simulink model "sinepwm"  (R2018a)
settings: Solver=VariableStepAuto  StartTime=0.0  StopTime=10  RelTol=1e-3
libraries: powerlib x21, simulink x7, powerlib_meascontrol x1
settings Model: Creator=Emre Deniz  LastModifiedBy=Emre Deniz
settings SolverCC: ZeroCrossAlgorithm=Adaptive
settings DebuggingCC: MaxConsecutiveZCsMsg=none

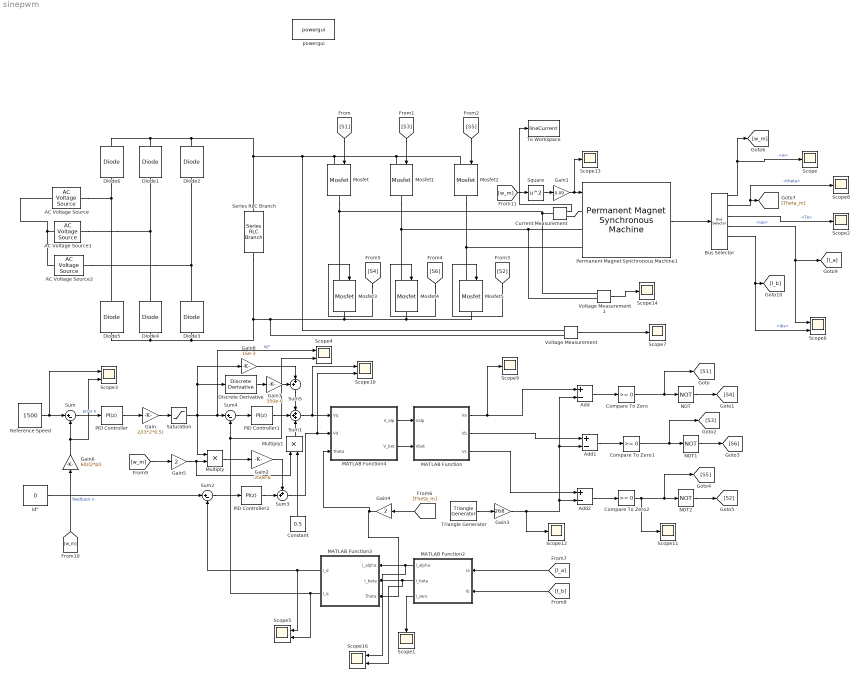
== system sinepwm ==
  AC Voltage Source : powerlib/Electrical Sources/AC Voltage Source  Amplitude=230*sqrt(2)  Phase=0  Frequency=50  SampleTime=0  Measurements=None  BusType=swing  Pref=10e3  Qref=0  Qmin=-inf  Qmax=+inf
  AC Voltage Source1 : powerlib/Electrical Sources/AC Voltage Source  Amplitude=230*sqrt(2)  Phase=-120  Frequency=50  SampleTime=0  Measurements=None  BusType=swing  Pref=10e3  Qref=0  Qmin=-inf  Qmax=+inf
  AC Voltage Source2 : powerlib/Electrical Sources/AC Voltage Source  Amplitude=230*sqrt(2)  Phase=+120  Frequency=50  SampleTime=0  Measurements=None  BusType=swing  Pref=10e3  Qref=0  Qmin=-inf  Qmax=+inf
  Add : Sum  Inputs=+-
  Add1 : Sum  Inputs=+-
  Add2 : Sum  Inputs=+-
  Bus Selector : BusSelector  OutputSignals=w,theta,Te,ias,ibs,ics
  Compare To Zero : simulink/Logic and Bit Operations/Compare To Zero  relop=>=  OutDataTypeStr=boolean
  Compare To Zero1 : simulink/Logic and Bit Operations/Compare To Zero  relop=>=  OutDataTypeStr=boolean
  Compare To Zero2 : simulink/Logic and Bit Operations/Compare To Zero  relop=>=  OutDataTypeStr=boolean
  Constant : Constant  Value=0.5
  Current Measurement : powerlib/Measurements/Current Measurement  PhasorSimulation=off  OutputType=Complex  PSBequivalent=0
  Diode{1..6} (6 alike) : powerlib/Power Electronics/Diode  Ron=0.001  Lon=0  Vf=0.8  IC=0  UseSnubber=0  Rs=500  Cs=250e-9  Measurements=off
  Discrete Derivative : simulink/Quick Insert/Discrete/Discrete Derivative  gainval=1.0  ICPrevScaledInput=0.0  OutMin=[]  OutMax=[]  OutDataType=fixdt(1, 16)  OutScaling=2^-10  DoSatur=off
      settings: SourceProductName=Simulink  SourceProductBaseCode=SL
  Gain : Gain  Gain=2/(3*2*0.5)
  Gain1 : Gain  Gain=0.09
  Gain2 : Gain  Gain=-350e-6
  Gain3 : Gain  Gain=268
  Gain4 : Gain  Gain=2
  Gain5 : Gain  Gain=2
  Gain6 : Gain  Gain=60/(2*pi)
  Gain7 : Gain  Gain=350e-6
  Gain8 : Gain  Gain=16e-3
  "Id\" " : Constant  Value=0
  MATLAB Function : MATLAB Function  TreatAsAtomicUnit=on
  MATLAB Function2 : MATLAB Function  TreatAsAtomicUnit=on
  MATLAB Function3 : MATLAB Function  TreatAsAtomicUnit=on
  MATLAB Function4 : MATLAB Function  TreatAsAtomicUnit=on
  Mosfet{,1..5} (6 alike) : powerlib/Power Electronics/Mosfet  Ron=0  Lon=0  Rd=0  Vfd=0  IC=0  Rs=1e9  Cs=inf  Measurements=off
  Multiply : Product
  Multiply1 : Product
  NOT : Logic  Operator=NOT  IconShape=distinctive  AllPortsSameDT=off  OutDataTypeStr=boolean
  NOT1 : Logic  Operator=NOT  IconShape=distinctive  AllPortsSameDT=off  OutDataTypeStr=boolean
  NOT2 : Logic  Operator=NOT  IconShape=distinctive  AllPortsSameDT=off  OutDataTypeStr=boolean
  PID Controller : simulink/Continuous/PID Controller  Controller=PI  TimeDomain=Discrete-time  SampleTime=-1  IntegratorMethod=Forward Euler  FilterMethod=Forward Euler  Form=Parallel  UseFilter=on  ControllerParametersSource=internal  P=200  I=1  D=0  N=100  InitialConditionSource=internal  InitialConditionForIntegrator=0  InitialConditionForFilter=0  ExternalReset=none  LimitOutput=off  UpperSaturationLimit=inf  LowerSaturationLimit=-inf  LinearizeAsGain=on  AntiWindupMode=none  Kb=1  TrackingMode=off  Kt=1  PParamMin=[]  PParamMax=[]  IParamMin=[]  IParamMax=[]  DParamMin=[]  DParamMax=[]  NParamMin=[]  NParamMax=[]  KbParamMin=[]  KbParamMax=[]  KtParamMin=[]  KtParamMax=[]  POutMin=[]  POutMax=[]  IOutMin=[]  IOutMax=[]  DOutMin=[]  DOutMax=[]  NOutMin=[]  NOutMax=[]  KbOutMin=[]  KbOutMax=[]  KtOutMin=[]  KtOutMax=[]  IntegratorOutMin=[]  IntegratorOutMax=[]  FilterOutMin=[]  FilterOutMax=[]  SumOutMin=[]  SumOutMax=[]  SumI1OutMin=[]  SumI1OutMax=[]  SumI2OutMin=[]  SumI2OutMax=[]  SumI3OutMin=[]  SumI3OutMax=[]  SumDOutMin=[]  SumDOutMax=[]  SaturationOutMin=[]  SaturationOutMax=[]  IntegratorContinuousStateAttributes=''  IntegratorStateMustResolveToSignalObject=off  IntegratorRTWStateStorageClass=Auto  FilterContinuousStateAttributes=''  FilterStateMustResolveToSignalObject=off  FilterRTWStateStorageClass=Auto  DifferentiatorICPrevScaledInput=0  DifferentiatorOutMin=[]  DifferentiatorOutMax=[]  FilterDiffOutCoefMin=[]  FilterDiffOutCoefMax=[]  SumDenOutMin=[]  SumDenOutMax=[]  SumNumOutMin=[]  SumNumOutMax=[]  ReciprocalOutMin=[]  ReciprocalOutMax=[]  DivideOutMin=[]  DivideOutMax=[]  TunerSelectOption=Transfer Function Based (PID Tuner App)
  PID Controller1 : simulink/Continuous/PID Controller  Controller=PI  TimeDomain=Discrete-time  SampleTime=-1  IntegratorMethod=Forward Euler  FilterMethod=Forward Euler  Form=Parallel  UseFilter=on  ControllerParametersSource=internal  P=0.01  I=50  D=0  N=100  InitialConditionSource=internal  InitialConditionForIntegrator=0  InitialConditionForFilter=0  ExternalReset=none  LimitOutput=off  UpperSaturationLimit=inf  LowerSaturationLimit=-inf  LinearizeAsGain=on  AntiWindupMode=none  Kb=1  TrackingMode=off  Kt=1  PParamMin=[]  PParamMax=[]  IParamMin=[]  IParamMax=[]  DParamMin=[]  DParamMax=[]  NParamMin=[]  NParamMax=[]  KbParamMin=[]  KbParamMax=[]  KtParamMin=[]  KtParamMax=[]  POutMin=[]  POutMax=[]  IOutMin=[]  IOutMax=[]  DOutMin=[]  DOutMax=[]  NOutMin=[]  NOutMax=[]  KbOutMin=[]  KbOutMax=[]  KtOutMin=[]  KtOutMax=[]  IntegratorOutMin=[]  IntegratorOutMax=[]  FilterOutMin=[]  FilterOutMax=[]  SumOutMin=[]  SumOutMax=[]  SumI1OutMin=[]  SumI1OutMax=[]  SumI2OutMin=[]  SumI2OutMax=[]  SumI3OutMin=[]  SumI3OutMax=[]  SumDOutMin=[]  SumDOutMax=[]  SaturationOutMin=[]  SaturationOutMax=[]  IntegratorContinuousStateAttributes=''  IntegratorStateMustResolveToSignalObject=off  IntegratorRTWStateStorageClass=Auto  FilterContinuousStateAttributes=''  FilterStateMustResolveToSignalObject=off  FilterRTWStateStorageClass=Auto  DifferentiatorICPrevScaledInput=0  DifferentiatorOutMin=[]  DifferentiatorOutMax=[]  FilterDiffOutCoefMin=[]  FilterDiffOutCoefMax=[]  SumDenOutMin=[]  SumDenOutMax=[]  SumNumOutMin=[]  SumNumOutMax=[]  ReciprocalOutMin=[]  ReciprocalOutMax=[]  DivideOutMin=[]  DivideOutMax=[]  TunerSelectOption=Transfer Function Based (PID Tuner App)
  PID Controller2 : simulink/Continuous/PID Controller  Controller=PI  TimeDomain=Discrete-time  SampleTime=-1  IntegratorMethod=Forward Euler  FilterMethod=Forward Euler  Form=Parallel  UseFilter=on  ControllerParametersSource=internal  P=0.01  I=20  D=0  N=100  InitialConditionSource=internal  InitialConditionForIntegrator=0  InitialConditionForFilter=0  ExternalReset=none  LimitOutput=off  UpperSaturationLimit=inf  LowerSaturationLimit=-inf  LinearizeAsGain=on  AntiWindupMode=none  Kb=1  TrackingMode=off  Kt=1  PParamMin=[]  PParamMax=[]  IParamMin=[]  IParamMax=[]  DParamMin=[]  DParamMax=[]  NParamMin=[]  NParamMax=[]  KbParamMin=[]  KbParamMax=[]  KtParamMin=[]  KtParamMax=[]  POutMin=[]  POutMax=[]  IOutMin=[]  IOutMax=[]  DOutMin=[]  DOutMax=[]  NOutMin=[]  NOutMax=[]  KbOutMin=[]  KbOutMax=[]  KtOutMin=[]  KtOutMax=[]  IntegratorOutMin=[]  IntegratorOutMax=[]  FilterOutMin=[]  FilterOutMax=[]  SumOutMin=[]  SumOutMax=[]  SumI1OutMin=[]  SumI1OutMax=[]  SumI2OutMin=[]  SumI2OutMax=[]  SumI3OutMin=[]  SumI3OutMax=[]  SumDOutMin=[]  SumDOutMax=[]  SaturationOutMin=[]  SaturationOutMax=[]  IntegratorContinuousStateAttributes=''  IntegratorStateMustResolveToSignalObject=off  IntegratorRTWStateStorageClass=Auto  FilterContinuousStateAttributes=''  FilterStateMustResolveToSignalObject=off  FilterRTWStateStorageClass=Auto  DifferentiatorICPrevScaledInput=0  DifferentiatorOutMin=[]  DifferentiatorOutMax=[]  FilterDiffOutCoefMin=[]  FilterDiffOutCoefMax=[]  SumDenOutMin=[]  SumDenOutMax=[]  SumNumOutMin=[]  SumNumOutMax=[]  ReciprocalOutMin=[]  ReciprocalOutMax=[]  DivideOutMin=[]  DivideOutMax=[]  TunerSelectOption=Transfer Function Based (PID Tuner App)
  Permanent Magnet Synchronous Machine1 : powerlib/Machines/Permanent Magnet Synchronous Machine  NbPhases=3  FluxDistribution=Sinusoidal  RotorType=Round  MechanicalLoad=Torque Tm  PresetModel=No  ShowDetailedParameters=on  MeasurementBus=on  Resistance=16e-3  Inductance=8.5e-3  dqInductances=[8.5e-3,8.5e-3]  La=350e-6  MachineConstant=Flux linkage established by magnets (V.s)  Flux=0.5  VoltageCst=181.3799  TorqueCst=1.5  Flat=120  Mechanical=[250 0 2 0]  PolePairs=4  InitialConditions=[141 ,0 ,0 ,0]  InitialConditions5ph=[0 0 0 0 0 0]  TsPowergui=0  TsBlock=-1  RefAngle=Aligned with phase A axis (original Park)
      settings: SourceProductName=Simscape Power Systems
  Reference Speed : Constant  Value=1500
  Saturation : Saturate  UpperLimit=1700  LowerLimit=-1700
  Scope{,1..2,7..9,11..14} (10 alike) : Scope
  Scope{3..6,10,16} (6 alike) : Scope  NumInputPorts=2
  Series RLC Branch : powerlib/Elements/Series RLC Branch  LConnTagsString=__new0  RConnTagsString=__new0  BranchType=C  Resistance=0.001  Inductance=1e-3  SetiL0=off  InitialCurrent=0  Capacitance=1  Setx0=on  InitialVoltage=540  Measurements=None
  Square : Math  Operator=square  SaturateOnIntegerOverflow=on
  Sum : Sum  Inputs=|+-
  Sum1 : Sum  Inputs=+++
  Sum2 : Sum  Inputs=|+-
  Sum3 : Sum  Inputs=++|
  Sum4 : Sum  Inputs=|+-
  Sum5 : Sum  Inputs=++|
  To Workspace : ToWorkspace  VariableName=lineCurrent  SaveFormat=Structure With Time  SampleTime=-1
  Triangle Generator : powerlib_meascontrol/Pulse & Signal Generators/Triangle Generator  Freq=3000  Phase=90  Ts=0
  Voltage Measurement : powerlib/Measurements/Voltage Measurement  PhasorSimulation=off  OutputType=Complex  PSBequivalent=0
  Voltage Measurement1 : powerlib/Measurements/Voltage Measurement  PhasorSimulation=off  OutputType=Complex  PSBequivalent=0
  powergui : powerlib/powergui  Priority=1  SimulationMode=Continuous  SampleTime=50e-6  frequency=60  Iterations=50  frequencyindice=50  Pbase=100e6  ErrMax=1e-4  UnitsV=kV  UnitsW=MW  buscounter=0  FunctionMessages=off  echomessages=off  EnableUseOfTLC=off  CurrentSourceSwitches=off  DisableSnubberDevices=off  DisableRonSwitches=off  DisableVfSwitches=off  DisplayEquations=off  SolverType=Tustin/Backward Euler (TBE)  Interpol=off  ExternalGateDelay=off  methode=off  Ts=100  x0status=blocks  SPID=on  SwTol=0  HookPort=off  RestoreLinks=warning  ResistiveCurrentMeasurement=off  Frange=[0:2:500]  Ylog=off  Xlog=on  ShowGrid=off  save=off  variable=ZData  structure=lineCurrent  ZoomFFT=off  StartTime=9.6  cycles=1  DisplayStyle=1  fundamental=50  FreqAxis=off  MaxFrequency=1000  frequencyindicesteady=1  RmsSteady=1  display=off
  wires:
  Reference Speed/1 -> Scope3/1, Sum/1
  [w_m] -> Gain6/1  "feedback n"
  Sum/1 -> PID Controller/1  "error n"
  PID Controller/1 -> Gain/1
  Gain/1 -> Saturation/1
  Saturation/1 -> Discrete Derivative/1, Gain8/1, Scope4/1, Sum4/1, Multiply/1  "iq*"
  PID Controller1/1 -> Sum1/2
  Sum1/1 -> MATLAB Function4/1(Vq), Scope10/1
  MATLAB Function4/1(V_alp) -> MATLAB Function/1(Valp)
  MATLAB Function4/2(V_bet) -> MATLAB Function/2(Vbet)
  MATLAB Function/1(Va) -> Scope9/1, Add/1
  MATLAB Function/2(Vb) -> Add1/1
  MATLAB Function/3(Vc) -> Add2/1
  MATLAB Function2/1(I_alpha) -> Scope16/1, MATLAB Function3/1(I_alpha)
  MATLAB Function2/2(I_beta) -> Scope16/2, MATLAB Function3/2(I_beta)
  MATLAB Function3/1(I_d) -> Scope5/1, Sum2/2
  "Id\" "/1 -> Sum2/1
  Sum2/1 -> PID Controller2/1
  PID Controller2/1 -> Sum3/2
  Sum3/1 -> MATLAB Function4/2(Vd), Scope10/2
  Multiply/1 -> Gain2/1
  Gain2/1 -> Sum3/1
  Sum4/1 -> PID Controller1/1
  MATLAB Function3/2(I_q) -> Scope5/2, Scope4/2, Sum4/2
  Add/1 -> Compare To Zero/1
  Add1/1 -> Compare To Zero1/1
  Add2/1 -> Compare To Zero2/1
  Triangle Generator/1 -> Gain3/1
  Compare To Zero/1 -> NOT/1, [S1]
  NOT/1 -> [S4]
  Gain3/1 -> Scope12/1, Add1/2, Add/2, Add2/2
  Compare To Zero1/1 -> NOT1/1, [S3]
  NOT1/1 -> [S6]
  Compare To Zero2/1 -> Scope11/1, NOT2/1, [S5]
  NOT2/1 -> [S2]
  [S1] -> Mosfet/1
  [S4] -> Mosfet3/1
  [S6] -> Mosfet4/1
  [S2] -> Mosfet5/1
  [S3] -> Mosfet1/1
  [S5] -> Mosfet2/1
  Permanent Magnet Synchronous Machine1/1 -> Bus Selector/1
  Bus Selector/1 -> Scope/1, [w_m]  "<w>"
  Bus Selector/2 -> Scope8/1, [Theta_m]  "<theta>"
  [Theta_m] -> Gain4/1
  Gain4/1 -> MATLAB Function4/3(Theta), MATLAB Function3/3(Theta)
  Bus Selector/4 -> Scope6/1, [I_a]  "<ias>"
  Bus Selector/5 -> Scope6/2, [I_b]  "<ibs>"
  [w_m] -> Gain5/1
  Gain5/1 -> Multiply1/1, Multiply/2
  Gain6/1 -> Scope3/2, Sum/2
  Multiply1/1 -> Sum1/3
  Constant/1 -> Multiply1/2
  [w_m] -> Square/1
  Square/1 -> Gain1/1
  Gain1/1 -> Scope13/1, Permanent Magnet Synchronous Machine1/1
  MATLAB Function2/3(I_zero) -> Scope1/1
  Bus Selector/3 -> Scope2/1  "<Te>"
  Voltage Measurement/1 -> Scope7/1
  Discrete Derivative/1 -> Gain7/1
  Gain7/1 -> Sum5/1
  Sum5/1 -> Sum1/1
  Gain8/1 -> Sum5/2
  Voltage Measurement1/1 -> Scope14/1
  Current Measurement/1 -> To Workspace/1
  [I_a] -> MATLAB Function2/1(Ia)
  [I_b] -> MATLAB Function2/2(Ib)
  connections:
  AC Voltage Source/RConn1 -- Diode5/RConn1 -- Diode6/LConn1
  Mosfet3/RConn1 -- Voltage Measurement/LConn2 -- Series RLC Branch/RConn1 -- Diode3/LConn1 -- Diode5/LConn1 -- Diode4/LConn1 -- Mosfet5/RConn1 -- Mosfet4/RConn1
  Mosfet2/LConn1 -- Voltage Measurement/LConn1 -- Diode2/RConn1 -- Diode1/RConn1 -- Diode6/RConn1 -- Series RLC Branch/LConn1 -- Mosfet/LConn1 -- Mosfet1/LConn1
  AC Voltage Source1/RConn1 -- Diode4/RConn1 -- Diode1/LConn1
  AC Voltage Source2/RConn1 -- Diode3/RConn1 -- Diode2/LConn1
  AC Voltage Source2/LConn1 -- AC Voltage Source/LConn1 -- AC Voltage Source1/LConn1
  Mosfet/RConn1 -- Current Measurement/LConn1 -- Voltage Measurement1/LConn1 -- Mosfet3/LConn1
  Mosfet1/RConn1 -- Voltage Measurement1/LConn2 -- Permanent Magnet Synchronous Machine1/LConn2 -- Mosfet4/LConn1
  Mosfet2/RConn1 -- Permanent Magnet Synchronous Machine1/LConn3 -- Mosfet5/LConn1
  Current Measurement/RConn1 -- Permanent Magnet Synchronous Machine1/LConn1

== matlab function sinepwm/MATLAB Function ==
  data: Valp input; Va output; Vbet input; Vb output; Vc output
function [Va,Vb,Vc] = invClarke(Valp,Vbet)

A = [ 1 0 1 ; -1/2 sqrt(3)/2 1 ; -1/2 -sqrt(3)/2 1];

Vo = 0;
Vin = [Valp;Vbet;Vo];

Vout = A* Vin;

Va = Vout(1);
Vb = Vout(2);
Vc = Vout(3);

== matlab function sinepwm/MATLAB Function2 ==
  data: Ia input; I_alpha output; Ib input; I_beta output; I_zero output
function [I_alpha, I_beta, I_zero] = Clarke(Ia,Ib)

Ic = - Ia - Ib;

A = (2/3)*[1 -1/2 -1/2 ; 0 sqrt(3)/2 -sqrt(3)/2 ; 1/2 1/2 1/2];

I_in = [Ia ; Ib; Ic];

I_out = A*I_in;

I_alpha = I_out(1);
I_beta = I_out(2);
I_zero = I_out(3);

== matlab function sinepwm/MATLAB Function3 ==
  data: I_alpha input; I_d output; I_beta input; I_q output; Theta input
function [I_d, I_q] = Park(I_alpha,I_beta,Theta)

I_in = [I_alpha ; I_beta];

A = [cos(Theta) sin(Theta) ; -sin(Theta) cos(Theta)];

I_out = A*I_in;

I_d = I_out(1);
I_q = I_out(2);

== matlab function sinepwm/MATLAB Function4 ==
  data: Vq input; V_alp output; Vd input; Theta input; V_bet output
function [V_alp, V_bet] = invPark(Vq,Vd,Theta)

A = [cos(Theta) -sin(Theta) ; sin(Theta) cos(Theta) ];


V = A* [Vd ; Vq];
V_alp = V(1);
V_bet = V(2);
